simulink model "LAB1__1_3"  (R2020a)
settings: Solver=VariableStepAuto  StartTime=0.0  StopTime=10.0  RelTol=1e-3
settings Model: Creator=Пользователь  LastModifiedBy=Пользователь

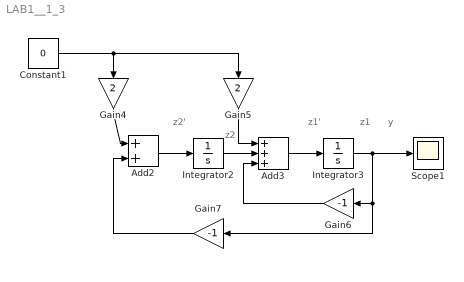
== system LAB1__1_3 ==
  note: z2'
  note: y
  note: z1
  note: z1'
  note: z2
  Add2 : Sum
  Add3 : Sum  Inputs=+++
  Constant1 : Constant  Value=0
  Gain4 : Gain  Gain=2
  Gain5 : Gain  Gain=2
  Gain6 : Gain  Gain=-1
  Gain7 : Gain  Gain=-1
  Integrator2 : Integrator  InitialCondition=0.5
  Integrator3 : Integrator  InitialCondition=1
  Scope1 : Scope
  wires:
  Integrator3/1 -> Gain6/1, Gain7/1, Scope1/1
  Constant1/1 -> Gain5/1, Gain4/1
  Integrator2/1 -> Add3/2
  Add2/1 -> Integrator2/1
  Gain4/1 -> Add2/1
  Gain7/1 -> Add2/2
  Gain6/1 -> Add3/3
  Gain5/1 -> Add3/1
  Add3/1 -> Integrator3/1
